simulink model "controller_for_carsimDIY"  (R2021a)
settings: Solver=VariableStepAuto  StartTime=0.0  StopTime=15  RelTol=1e-2
libraries: Solver_SF x1, simulink_extras x1, simulink x1
settings Model: Creator=dekunw  LastModifiedBy=chnwa
settings SolverCC: AlgebraicLoopSolver=LineSearch
settings DebuggingCC: SFMachineParentedDataDiag=warning

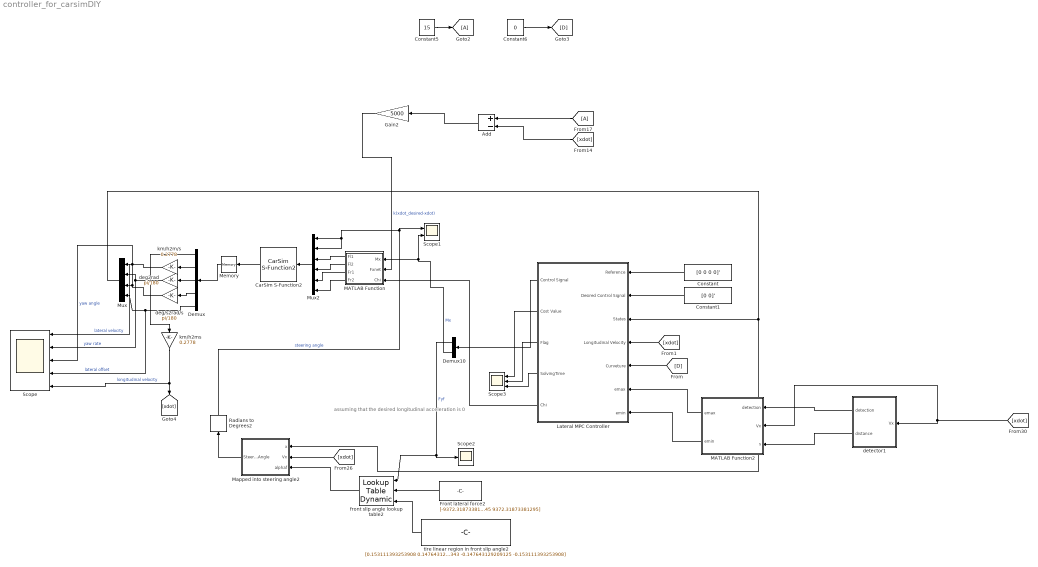
== system controller_for_carsimDIY ==
  note: assuming that the desired longitudinal acceleration is 0
  Add : Sum  Inputs=+-
  CarSim S-Function2 : Solver_SF/CarSim S-Function2  Priority=1  VehicleCode=i_i  SIMFILE=simfile.sim
      settings: AttributesFormatString=Vehicle Code: %<VehicleCode>
  Constant : Constant  Value=[0 0 0 0]'
  Constant1 : Constant  Value=[0 0]'
  Constant5 : Constant  Value=15
  Constant6 : Constant  Value=0
  Demux : Demux  Outputs=5
  Demux10 : Demux  Outputs=2
  Front lateral force2 : Constant  Value="[-9372.31873381295\t-9371.87234490745\t-9368.75632133124\t-9360.32413915416\t-9343.95286497491\t-9317.04140044534\t-9277.00875557097\t-9221.29234898623\t-9147.34633344744\t-9052.63994482675\t-8934.65587292915\t-8790.88865249026\t-8618.84307274575\t-8416.03260399439\t-8179.97783960505\t-7908.20495194422\t-7598.24416072470\t-7247.62821229778\t-6853.89086843106\t-6414.56540313147\t-5927.18310608872\t-5389.27179132790\t-4798.35430967129\t-4151.94706361935\t-3447.55852326814\t-2682.68774188626\t-1854.82286977838\t-961.439665063923\t0\t961.439665063923\t1854.82286977838\t2682.68774188626\t3447.55852326814\t4151.94706361935\t4798.35430967129\t5389.27179132790\t5927.18310608872\t6414.56540313147\t6853.89086843106\t7247.62821229778\t7598.24416072470\t7908.20495194422\t8179.97783960505\t8416.03260399439\t8618.84307274575\t8790.88865249026\t8934.65587292915\t9052.63994482675\t9147.34633344744\t9221.29234898623\t9277.00875557097\t9317.04140044534\t9343.95286497491\t9360.32413915416\t9368.75632133124\t9371.87234490745\t9372.31873381295]"
  Gain2 : Gain  Gain=5000
  Lateral MPC Controller : Subsystem
  MATLAB Function : MATLAB Function  TreatAsAtomicUnit=on
  MATLAB Function2 : MATLAB Function  TreatAsAtomicUnit=on
  Mapped into steering angle2 : MATLAB Function  TreatAsAtomicUnit=on
  Memory : Memory  InitialCondition=[54 0 0 0 0]'
  Mux : Mux
  Mux2 : Mux  Inputs=6
  Radians to Degrees2 : simulink_extras/Transformations/Radians to Degrees
  Scope : Scope  NumInputPorts=5
  Scope1 : Scope  NumInputPorts=2
  Scope2 : Scope
  Scope3 : Scope  NumInputPorts=3
  deg/s2rad/s : Gain  Gain=pi/180
  deg2rad : Gain  Gain=pi/180
  detector1 : Subsystem
  front slip angle lookup table2 : simulink/Lookup Tables/Lookup Table Dynamic  LookUpMeth=Interpolation-Use End Values  OutDataType=fixdt('double')  OutScaling=[]  OutputDataTypeScalingMode=Specify via dialog  OutDataTypeStr=double  DoSatur=off
  km/h2m/s : Gain  Gain=0.2778
  km/h2ms : Gain  Gain=0.2778
  tire linear region in front slip angle2 : Constant  Value="[0.153111393253908\t0.147643129209125\t0.142174865164343\t0.136706601119560\t0.131238337074778\t0.125770073029996\t0.120301808985213\t0.114833544940431\t0.109365280895648\t0.103897016850866\t0.0984287528060835\t0.0929604887613011\t0.0874922247165187\t0.0820239606717363\t0.0765556966269539\t0.0710874325821714\t0.0656191685373890\t0.0601509044926066\t0.0546826404478242\t0.0492143764030418\t0.0437461123582594\t0.0382778483134769\t0.0328095842686945\t0.0273413202239121\t0.0218730561791297\t0.0164047921343473\t0.0109365280895648\t0.00546826404478242\t0\t-0.00546826404478242\t-0.0109365280895648\t-0.0164047921343473\t-0.0218730561791297\t-0.0273413202239121\t-0.0328095842686945\t-0.0382778483134769\t-0.0437461123582594\t-0.0492143764030418\t-0.0546826404478242\t-0.0601509044926066\t-0.0656191685373890\t-0.0710874325821714\t-0.0765556966269539\t-0.0820239606717363\t-0.0874922247165187\t-0.0929604887613011\t-0.0984287528060835\t-0.103897016850866\t-0.109365280895648\t-0.114833544940431\t-0.120301808985213\t-0.125770073029996\t-0.131238337074778\t-0.136706601119560\t-0.142174865164343\t-0.147643129209125\t-0.153111393253908]"
  wires:
  [xdot] -> MATLAB Function2/2(Vx), detector1/1(Vx)
  Demux10/2 -> Scope1/2, MATLAB Function/1(Mx)  "Mx"
  tire linear region in front slip angle2/1 -> front slip angle lookup table2/3
  [xdot] -> Mapped into steering angle2/2(Vx)
  Demux10/1 -> Scope2/1, front slip angle lookup table2/1  "Fyf"
  Front lateral force2/1 -> front slip angle lookup table2/2
  [xdot] -> Add/2
  [A] -> Add/1
  Add/1 -> Gain2/1
  Gain2/1 -> MATLAB Function/2(Fxnet)  "k(xdot_desired-xdot)"
  Radians to Degrees2/1 -> Mux2/2, Mux2/1, Scope1/1  "steering angle"
  front slip angle lookup table2/1 -> Mapped into steering angle2/3(alphaf)
  Mapped into steering angle2/1(SteeringAngle) -> Radians to Degrees2/1
  Constant5/1 -> [A]
  Constant6/1 -> [D]
  Demux/1 -> km/h2ms/1
  km/h2m/s/1 -> Scope/1, Mux/1  "lateral velocity"
  deg2rad/1 -> Scope/2, Mux/2  "yaw rate"
  Demux/4 -> deg/s2rad/s/1
  Demux/5 -> Scope/4, Mux/4  "lateral offset"
  Mux2/1 -> CarSim S-Function2/1
  CarSim S-Function2/1 -> Memory/1
  km/h2ms/1 -> [xdot], Scope/5  "longitudinal velocity"
  Demux/2 -> km/h2m/s/1
  Demux/3 -> deg2rad/1
  deg/s2rad/s/1 -> Scope/3, Mux/3  "yaw angle"
  MATLAB Function/1(Fl1) -> Mux2/3
  MATLAB Function/2(Fl2) -> Mux2/4
  MATLAB Function/3(Fr1) -> Mux2/5
  MATLAB Function/4(Fr2) -> Mux2/6
  Lateral MPC Controller/4(SolvingTime) -> Scope3/3
  Lateral MPC Controller/3(Flag) -> Scope3/2
  Lateral MPC Controller/2(Cost Value) -> Scope3/1
  Lateral MPC Controller/1(Control Signal) -> Demux10/1
  Constant/1 -> Lateral MPC Controller/1(Reference)
  Constant1/1 -> Lateral MPC Controller/2(Desired Control Signal)
  [D] -> Lateral MPC Controller/5(Curveture)
  MATLAB Function2/2(emin) -> Lateral MPC Controller/7(emin)
  MATLAB Function2/1(emax) -> Lateral MPC Controller/6(emax)
  [xdot] -> Lateral MPC Controller/4(Longitudinal Velocity)
  Mux/1 -> Mapped into steering angle2/1(x), Lateral MPC Controller/3(States)
  Memory/1 -> Demux/1
  detector1/2(distance) -> MATLAB Function2/3(s)
  detector1/1(detection) -> MATLAB Function2/1(detection)
  Lateral MPC Controller/5(Chi) -> MATLAB Function/3(Chi)

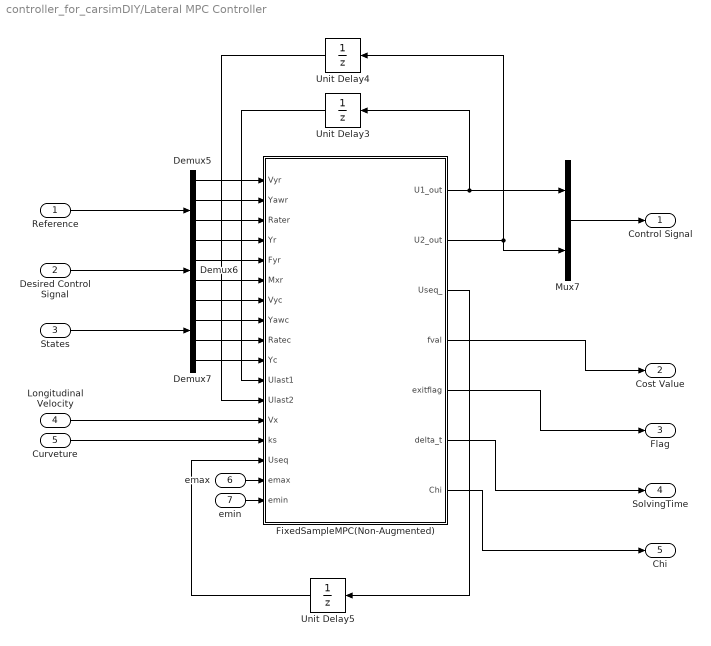
== system controller_for_carsimDIY/Lateral MPC Controller ==
  Reference : Inport
  Desired Control Signal : Inport  Port=2
  States : Inport  Port=3
  Longitudinal Velocity : Inport  Port=4
  Curveture : Inport  Port=5
  emax : Inport  Port=6
  emin : Inport  Port=7
  Demux5 : Demux
  Demux6 : Demux  Outputs=2
  Demux7 : Demux
  FixedSampleMPC(Non-Augmented) : MATLAB Function  TreatAsAtomicUnit=on
  Mux7 : Mux  Inputs=2
  Unit Delay3 : UnitDelay  SampleTime=-1  HasFrameUpgradeWarning=on
  Unit Delay4 : UnitDelay  SampleTime=-1  HasFrameUpgradeWarning=on
  Unit Delay5 : UnitDelay  InitialCondition=zeros(31,2)  SampleTime=-1  HasFrameUpgradeWarning=on
  Control Signal : Outport
  Cost Value : Outport  Port=2
  Flag : Outport  Port=3
  SolvingTime : Outport  Port=4
  Chi : Outport  Port=5
  wires:
  Demux5/3 -> FixedSampleMPC(Non-Augmented)/3(Rater)
  Desired Control Signal/1 -> Demux6/1
  FixedSampleMPC(Non-Augmented)/5(exitflag) -> Flag/1
  FixedSampleMPC(Non-Augmented)/2(U2_out) -> Mux7/2, Unit Delay4/1
  Demux5/1 -> FixedSampleMPC(Non-Augmented)/1(Vyr)
  Unit Delay4/1 -> FixedSampleMPC(Non-Augmented)/12(Ulast2)
  Longitudinal Velocity/1 -> FixedSampleMPC(Non-Augmented)/13(Vx)
  Demux7/3 -> FixedSampleMPC(Non-Augmented)/9(Ratec)
  FixedSampleMPC(Non-Augmented)/3(Useq_) -> Unit Delay5/1
  Demux7/1 -> FixedSampleMPC(Non-Augmented)/7(Vyc)
  Demux5/4 -> FixedSampleMPC(Non-Augmented)/4(Yr)
  FixedSampleMPC(Non-Augmented)/4(fval) -> Cost Value/1
  Curveture/1 -> FixedSampleMPC(Non-Augmented)/14(ks)
  emax/1 -> FixedSampleMPC(Non-Augmented)/16(emax)
  FixedSampleMPC(Non-Augmented)/1(U1_out) -> Mux7/1, Unit Delay3/1
  Demux7/2 -> FixedSampleMPC(Non-Augmented)/8(Yawc)
  Demux7/4 -> FixedSampleMPC(Non-Augmented)/10(Yc)
  Reference/1 -> Demux5/1
  Mux7/1 -> Control Signal/1
  Unit Delay5/1 -> FixedSampleMPC(Non-Augmented)/15(Useq)
  Unit Delay3/1 -> FixedSampleMPC(Non-Augmented)/11(Ulast1)
  States/1 -> Demux7/1
  FixedSampleMPC(Non-Augmented)/6(delta_t) -> SolvingTime/1
  Demux6/2 -> FixedSampleMPC(Non-Augmented)/6(Mxr)
  Demux6/1 -> FixedSampleMPC(Non-Augmented)/5(Fyr)
  Demux5/2 -> FixedSampleMPC(Non-Augmented)/2(Yawr)
  emin/1 -> FixedSampleMPC(Non-Augmented)/17(emin)
  FixedSampleMPC(Non-Augmented)/7(Chi) -> Chi/1

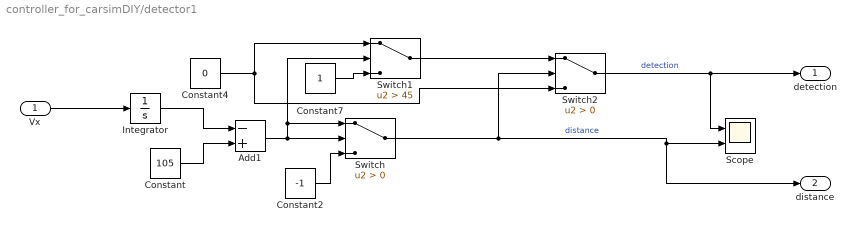
== system controller_for_carsimDIY/detector1 ==
  Vx : Inport
  Add1 : Sum  Inputs=-+
  Constant : Constant  Value=105
  Constant2 : Constant  Value=-1
  Constant4 : Constant  Value=0
  Constant7 : Constant
  Integrator : Integrator
  Scope : Scope  NumInputPorts=2
  Switch : Switch  Criteria=u2 > Threshold
  Switch1 : Switch  Criteria=u2 > Threshold  Threshold=45
  Switch2 : Switch  Criteria=u2 > Threshold
  detection : Outport
  distance : Outport  Port=2
  wires:
  Constant2/1 -> Switch/3
  Constant4/1 -> Switch2/3, Switch1/1
  Vx/1 -> Integrator/1
  Integrator/1 -> Add1/1
  Switch/1 -> Switch2/2, Scope/2, distance/1  "distance"
  Constant7/1 -> Switch1/3
  Add1/1 -> Switch1/2, Switch/1, Switch/2
  Switch1/1 -> Switch2/1
  Constant/1 -> Add1/2
  Switch2/1 -> Scope/1, detection/1  "detection"

== matlab function controller_for_carsimDIY/MATLAB Function2 ==
  data: detection input; Vx input size=1; s input; emax output; emin output
function [emax,emin] = fcn(detection,Vx,s)
PredictionHorizon=30;
Ts=0.1;
k = round(s/Vx/Ts);
if k>PredictionHorizon
    k =PredictionHorizon;
elseif k<20
    k=20;
end

if detection == 1
    emin = -10*ones(PredictionHorizon,1);
    emax=   10*ones(PredictionHorizon,1);
    k1=k-round(3/Vx/Ts);
    k2=k+round(3/Vx/Ts);
    if k1<1
        k1=1;
    end
    if k2>PredictionHorizon
        k2=PredictionHorizon;
    end
    emin(k1:k2)=4;
    emax(k1:k2)=6;
else
    emin=-10*ones(PredictionHorizon,1);
    emax=10*ones(PredictionHorizon,1);
end

== matlab function controller_for_carsimDIY/Lateral MPC Controller/FixedSampleMPC(Non-Augmented) ==
  data: Vyr input; U1_out output; Yawr input; Rater input; Yr input; Fyr input; Mxr input; Vyc input; Yawc input; Ratec input; Yc input; Ulast1 input; Ulast2 input; Vx input; ks input; Useq input; U2_out output; Useq_ output; fval output; exitflag output; delta_t output; emax input; emin input; Chi output
function [U1_out,U2_out,Useq_,fval,exitflag,delta_t,Chi] = fcn(Vyr,Yawr,Rater,Yr, Fyr,Mxr,Vyc,Yawc,Ratec,Yc,Ulast1,Ulast2,Vx,ks,Useq,emax,emin)
%Vyr lateral velocity, Yawr yaw angle, Rater yaw rate, Yr lateral position
%Fyr lateral force in front tyre,Mxr moment generated by longitudinal force
%'r'means reference ||  'c'means current
    if Vx<0.1
        Vx=0.001;%make sure many expressions' denominator isn't 0
    end
    lr=1.67;
    threshold=0.1022; %largest rear slip angle in linear region
    miu=0.7;
    rmax=9.81*miu/Vx;
%% Initilization    
    tstart=tic;%timing on
    
    Nx=4;%number of state
    Nu=2;%number of control
    Np=30;%prediction horizon
    Nc=1;%control horizon

    %reference
    r=zeros(Nx,1);%state reference
    r(1)=Vyr;
    r(2)=Yawr;
    r(3)=Rater;
    r(4)=Yr;    
    ur1=Fyr;
    ur2=Mxr;%control reference
    
    %states
    x=zeros(Nx,1);%state reference
    x(1)=Vyc;
    x(2)=Yawc;
    x(3)=Ratec;
    x(4)=Yc;   
    
    %control
    u=zeros(Nu,1);%state reference
    u(1)=Ulast1;
    u(2)=Ulast2;
    
    %get augmented states
    kesi=zeros(Nx+Nu,1);%[X;U]
    kesi(1)=x(1)-r(1);
    kesi(2)=x(2)-r(2);
    kesi(3)=x(3)-r(3);
    kesi(4)=x(4)-r(4);
    kesi(5)=u(1)-ur1;
    kesi(6)=u(2)-ur2;
    
    Ts=0.05;%sample time
    
%% Modellng->Discretization->prediction->quadratic programming
    %Modelling&Linearization&Discretization
    steps=Np+1;
    A = zeros(Nx+Nu,Nx+Nu,steps);
    B = zeros(Nx+Nu,Nu,steps);
    Dc = zeros(Nx+Nu,1,steps);
    C=[1 0 0 0 0 0;0 1 0 0 0 0;0 0 1 0 0 0;0 0 0 1 0 0];
    
    for ct = 1:steps
        if ct>length(Useq)
            uk = Useq(Np,:);
        else
            uk = Useq(ct,:);
        end
        uk=uk';
        [Ad, Bd, DK, delta_x] = GetDynamics(Vx,ks,x,uk,Ts);
        A(:,:,ct)=[Ad,Bd;zeros(Nu,Nx),eye(Nu)];        
        B(:,:,ct)=[Bd;eye(Nu)];
        Dc(:,:,ct)=[DK;0;0];
        x=x+delta_x;    
    end
    %construct important matrix
    %Y=PHI*kesi+THETA*delta_U+OMEGA*D
    coder.varsize('PHI',[Np*Nx,Nx+Nu]);
    coder.varsize('THETA',[Np*Nx,Nc*Nu]);
    coder.varsize('D',[Np*(Nx+Nu),1]);
    coder.varsize('DD',[Np*Nx,1]);
    PHI=[];
    THETA=[];
    D=[];
    DD=[];
    product=eye(6);
    for j=1:Np
        product=A(:,:,j)*product;
        PHI=[PHI;C*product];
        D=[D;Dc(:,:,j)];
    end
    for k=1:Nc
        product1=eye(6);
        for j=1:Np
            THETA=[THETA;C*product1*B(:,:,k)];
            product1=A(:,:,j+1)*product1;
        end
    end
    coder.varsize('OMEGA',[Nx*Np,(Nx+Nu)*Np]);
    OMEGA=zeros(Nx*Np,(Nx+Nu)*Np);
    for i=1:Np
        product2=A(:,:,i+1);
        for j=i:Np-1
            if i==j
                OMEGA(4*i-3:4*i,6*i-5:6*i)=C*eye(6);
            end
            OMEGA(4*j+1:4*j+4,6*j+1:6*j+6)=C*product2;
            product2=A(:,:,j+2)*product2;
        end
    end
    DD=OMEGA*D;        
    Sigma=zeros(Np,Nc);
    for p=1:Np%define a lower triangular matrix
        for q=1:1:Nc
            if q<=p 
                Sigma(p,q)=1;
            else 
                Sigma(p,q)=0;
            end
        end 
    end 
    UT=kron(ones(Np,1),[u(1);u(2)]);
    Sigma=kron(Sigma,eye(Nu));
    error=PHI*kesi;
    Q=kron(eye(Np,Np),diag([0 0 100 4]));    
    R=kron(eye(Np,Np),diag([0 4e-5]));    
    P=diag([3e-5 8e-5]);
    rou1=3e3;    
    rou2=5e4;
    H=2*[THETA'*Q*THETA+Sigma'*R*Sigma+P zeros(2,2);0 0 rou1 0;0 0 0 rou2];%是否要乘2？要
    f=[2*(error'*Q*THETA+(OMEGA*D)'*Q*THETA+UT'*R*Sigma),0,0];%是否要转置？好像无所谓
   %% constraints
    if abs(x(2))<=rmax
        Chi1=1;
    elseif abs(x(2))>rmax&&abs(x(2))<=(1+0.1)*rmax
        Chi1=1-(abs(x(2)-rmax))/(0.1*rmax);
    else
        Chi1=0;
    end
    alphar=(x(1)-lr*x(2))/Vx; %alphar is the slip angle of rear tyre
    if abs(alphar)<=threshold
        Chi2=1;
    elseif abs(alphar)>threshold&&abs(alphar)<=(1+0.1)*threshold
        Chi2=1-(abs(alphar)-threshold)/(0.1*threshold);
    else
        Chi2=0;
    end
    Chi=min(Chi1,Chi2);%Chi adjusts the max allowable moments generated by longitudinal forces, lower it as it moves out of the parrallelogram
    %inequation
    A_t=zeros(Nc,Nc);
    for p=1:1:Nc%define a lower triangular matrix
        for q=1:1:Nc
            if q<=p 
                A_t(p,q)=1;
            else 
                A_t(p,q)=0;
            end
        end 
    end 
    A_I=kron(A_t,eye(Nu)); 
    Ut=kron(ones(Nc,1),[Ulast1;Ulast2]);%control in last control step
    umin=[-1e4; -1e3*Chi];
    umax=[1e4; 1e3*Chi];
    Umin=kron(ones(Nc,1),umin);
    Umax=kron(ones(Nc,1),umax);
    coder.varsize('A_cons',[Np*6+4,4]);
    coder.varsize('b_cons',[Np*6+4,1]);
    A_cons=[A_I zeros(Nu*Nc,2);-A_I zeros(Nu*Nc,2)];
    b_cons=[Umax-Ut;-Umin+Ut];
    %add handling envelop constriants & environment envolop
    gamas=[1 -lr 0 0;-1 lr 0 0;0 1 0 0;0 -1 0 0];
    gamae=[0 0 0 1;0 0 0 -1];
    Gs=[Vx*threshold;Vx*threshold;rmax;rmax];
    for i=1:Np
        A_cons=[A_cons;[gamas*THETA(4*i-3:4*i,:) -ones(4,1) zeros(4,1)];[gamae*THETA(4*i-3:4*i,:) zeros(2,1) -ones(2,1)]];
        b_cons=[b_cons;[Gs-gamas*(PHI(4*i-3:4*i,:)*kesi-DD(4*i-3:4*i,:))];[emax(i);-emin(i)]-gamae*(PHI(4*i-3:4*i,:)*kesi-DD(4*i-3:4*i,:))];
    end
    
    %upper and lower boundary
    delta_umin=[-1e4;-1e3];
    delta_umax=[1e4;1e3];
    M1=10; %related to slack variable
    M2=10; %related to slack variable
    delta_Umin=kron(ones(Nc,1),delta_umin);
    delta_Umax=kron(ones(Nc,1),delta_umax);
    lb=[delta_Umin;0;0];
    ub=[delta_Umax;M1;M2];  
   %% solve quadratic programming
    opts = optimoptions('quadprog','Algorithm','active-set');
    x_start=zeros(Nu*Nc+2,1);%+2 corresponds to slack variables
    [X,fval,exitflag]=quadprog(H,f',A_cons,b_cons,[],[],lb,ub,x_start,opts);
    
   %% calculate control signal
    U1=kesi(5)+X(1);%The output error at the previous time plus the optimization result to get the error at this time
    U2=kesi(6)+X(2);%The output error at the previous time plus the optimization result to get the error at this time
    U1_out=U1+ur1;%Error plus reference value to get final output value    
    U2_out=U2+ur2;
    Useq_=repmat([U1,U2],Np+1,1); %adaptive MPC block's method
%     Useq_=[[U1,U2];repmat(zeros(1,2),Np,1)]; %this may make more sense
    delta_t=toc(tstart);%timing off
end

function [A, B, DK, delta_x] = GetDynamics(Vx,ks,x,u,Ts)

%Plant Model parameters
m = 2272;   %mass
Iz = 4600;  %rotational inertia
lf = 1.11;  % distance from front axle to the mass center
lr = 1.67;  % distance from rear axle to the mass center
C_a = 1.822e5; % rear cornering stiffness 

%Enviroment parameters
miu = 0.7; %frction cooeficient 0.7 for dry road and 0.4 for wet
g = 9.81; % gravity

Fz = m*g*lf/(lf+lr); % the load that beared by the rear tire

%calculate alpha
Vy = x(1); %lateral velocity
r = x(2);  %yaw rate
alphar_ = Vy/Vx-lr*r/Vx;   %calculate linearzing point

%tire model
threshold = atan(3*miu*Fz/C_a);     % threshold for the tire linear region
if abs(alphar_)<threshold
    %the rear lateral force value (f(x0)) at the linearzing point
    Fyr_ = -C_a*tan(alphar_)+C_a^2/(3*miu*Fz)*abs(tan(alphar_))*tan(alphar_)-C_a^3/(27*miu^2*Fz^2)*tan(alphar_)^3;
    
    %the slope of linearized model (f‘(x0))
    if alphar_>= 0
        Cr_ = -C_a*sec(alphar_)^2+C_a^2/(3*miu*Fz)*(2*sec(alphar_)^2*tan(alphar_))-C_a^3/(27*miu^2*Fz^2)*(3*tan(alphar_)^2*sec(alphar_)^2);
    else
        Cr_ = -C_a*sec(alphar_)^2-C_a^2/(3*miu*Fz)*(2*sec(alphar_)^2*tan(alphar_))-C_a^3/(27*miu^2*Fz^2)*(3*tan(alphar_)^2*sec(alphar_)^2);
    end
else
    
    %the saturation region of tire model
    Fyr_ = -miu*Fz*sign(alphar_);
    Cr_ = 0;
end

%Continuous-time model
Ac = [Cr_/(m*Vx) -lr*Cr_/(m*Vx)-Vx 0 0;
    -lr*Cr_/(Iz*Vx) lr^2*Cr_/(Iz*Vx) 0 0;
    0 1 0 0;
    1 0 Vx 0];
Bc = [1/m 0;
    lf/Iz 1/Iz;
    0 0;
    0 0];
dcc = [(Fyr_-Cr_*alphar_)/m;
    -lr*(Fyr_-Cr_*alphar_)/Iz;
    -Vx*ks;
    0];

G=[Ac Bc dcc;zeros(3,7)];
M=expm(G*Ts);
A=M(1:4,1:4);
B=M(1:4,5:6);
DK=M(1:4,7);
delta_x=A*x+B*u+DK-x;
end

== matlab function controller_for_carsimDIY/Mapped into steering angle2 ==
  data: x input; Vx input; alphaf input; SteeringAngle output
function SteeringAngle = fcn(x,Vx, alphaf)

lf = 1.11;  % distance from front axle to the mass center

Vy = x(1); %lateral velocity
r = x(2);  %yaw rate
SteeringAngle = Vy/Vx+lf*r/Vx-alphaf;

== matlab function controller_for_carsimDIY/MATLAB Function ==
  data: Fl1 output; Mx input; Fl2 output; Fxnet input; Fr1 output; Fr2 output; Chi input
function [Fl1,Fl2,Fr1,Fr2] = fcn(Mx,Fxnet,Chi)
Eta_e=0.5; % the ratio of the allocated brakes on the front axle when Chi=1
Eta_f=0.7; % the ratio of the allocated brakes on the front axle when Chi=0
Eta=Eta_f-Chi*(Eta_f-Eta_e);
w = 1.875; % the width of the car

Fwf = zeros(2,1);
Fwr = zeros(2,1);

if Mx > 0
    Fwf(1) = Fxnet/2+0;
    Fwf(2) = Fxnet/2-Eta*2*Mx/w;
    Fwr(1) = 0;
    Fwr(2) = -(1-Eta)*2*Mx/w;
elseif Mx < 0
    Fwf(1) = Fxnet/2+Eta*2*Mx/w;
    Fwf(2) = Fxnet/2+0;
    Fwr(1) = (1-Eta)*2*Mx/w;
    Fwr(2) = 0;
else
    Fwf(1) = Fxnet/2+0;
    Fwf(2) = Fxnet/2+0;
    Fwr(1) = 0;
    Fwr(2) = 0;
end
Fl1 = Fwf(1);
Fl2 = Fwr(1);
Fr1 = Fwf(2);
Fr2 = Fwr(2);
